simulink model "Satellite_formation_control_stable_consensus"  (R2022b)
settings: Solver=VariableStepAuto  StartTime=0.0  StopTime=500  RelTol=1e-3
values from neighbouring files (symbols this model uses):
  Am = kron(eye(N),A)    [Robust_consensus.m]    (also in Robust_consensus_S_procedure.m = blkdiag(A,(1+delta2)*A, (1+delta3)*A, (1+delta4)*A, (1+delta; Robust_consensus_against_model_uncertainty.m = blkdiag(A,A+Delta2, A+Delta3, A+Delta4, A+Delta5, A+Delta6); Stable_Consensus.m; alpha_stability.m = blkdiag(A,A+Delta2, A+Delta3, A+Delta4, A+Delta5, A+Delta6))
  Bm = kron(eye(N),B)    [Robust_consensus.m]    (also in Robust_consensus_S_procedure.m; Robust_consensus_against_model_uncertainty.m; Stable_Consensus.m; alpha_stability.m)
  Cm = kron(eye(N),C)    [output_feedback_formation_control.m]
  Km = kron(L,-c*B*K)    [Robust_consensus.m]    (also in Robust_consensus_S_procedure.m; Robust_consensus_against_model_uncertainty.m; Stable_Consensus.m; alpha_stability.m = kron(L,c*B*K))
  x0 = [x1_0 ... (first row only)    [Robust_consensus.m]    (also in Robust_consensus_S_procedure.m; Robust_consensus_against_model_uncertainty.m; Stable_Consensus.m; alpha_stability.m)
  x1_0 = [0 500 866*sqrt(3) 1.5 0 0].'    [Robust_consensus.m]    (also in Robust_consensus_S_procedure.m; Robust_consensus_against_model_uncertainty.m; Stable_Consensus.m; alpha_stability.m)
  xd = [x1d ... (first row only)    [Robust_consensus.m]    (also in Robust_consensus_S_procedure.m; Robust_consensus_against_model_uncertainty.m; Stable_Consensus.m; alpha_stability.m)
settings Model: Creator=yu zheng  LastModifiedBy=Abelb
settings SolverCC: AlgebraicLoopSolver=TrustRegion
settings DebuggingCC: UnconnectedInputMsg=warning  UnconnectedOutputMsg=warning  UnconnectedLineMsg=warning  SFMachineParentedDataDiag=warning
settings ModelReferenceCC: EnableRefExpFcnMdlSchedulingChecks=on
settings RTWCC: DLArmComputeVersion=19.05

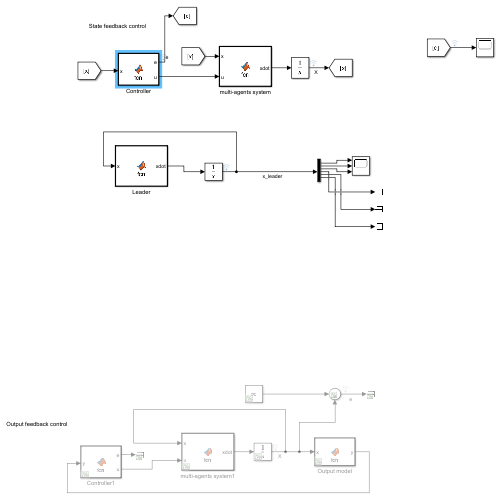
[thumbnail: Simulink's stored preview of the top-level diagram]
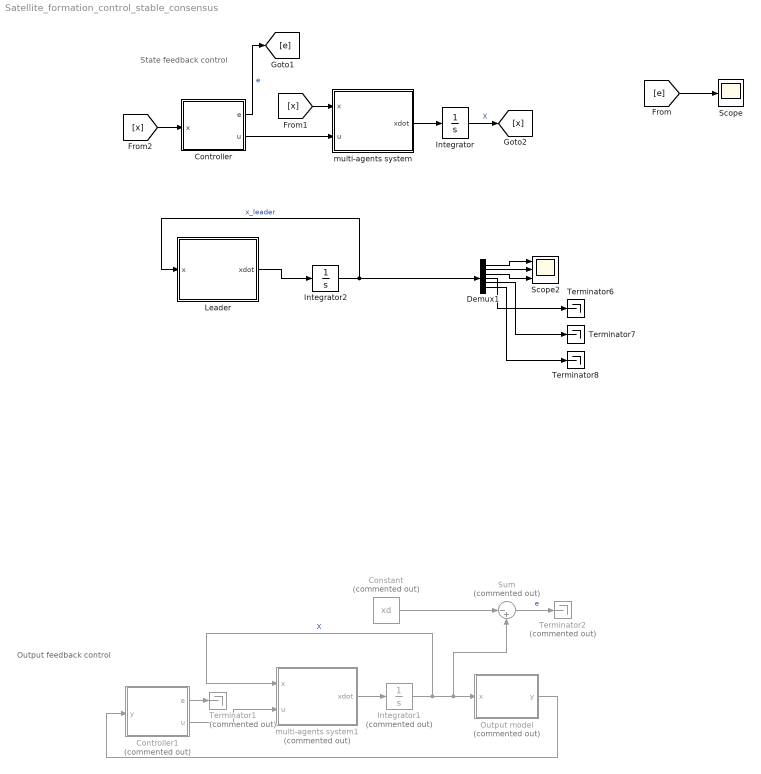
== system Satellite_formation_control_stable_consensus ==
  note: State feedback control
  note: Output feedback control
  Constant : Constant  Commented=on  Value=xd
  Controller : MATLAB Function  TreatAsAtomicUnit=on
  Controller1 : MATLAB Function  Commented=on  TreatAsAtomicUnit=on
  Demux1 : Demux  Outputs=6
  Integrator : Integrator  InitialCondition=x0
  Integrator1 : Integrator  Commented=on  InitialCondition=x0
  Integrator2 : Integrator  InitialCondition=x1_0
  Leader : MATLAB Function  TreatAsAtomicUnit=on
  Output model : MATLAB Function  Commented=on  TreatAsAtomicUnit=on
  Scope : Scope
  Scope2 : Scope  NumInputPorts=3
  Sum : Sum  Commented=on  Inputs=|-+
  Terminator1 : Terminator  Commented=on
  Terminator2 : Terminator  Commented=on
  Terminator6 : Terminator
  Terminator7 : Terminator
  Terminator8 : Terminator
  multi-agents system : MATLAB Function  TreatAsAtomicUnit=on
  multi-agents system1 : MATLAB Function  Commented=on  TreatAsAtomicUnit=on
  wires:
  multi-agents system/1(xdot) -> Integrator/1
  Integrator/1 -> [x]  "X"
  Controller/2(u) -> multi-agents system/2(u)
  Controller/1(e) -> [e]  "e"
  multi-agents system1/1(xdot) -> Integrator1/1
  Controller1/2(u) -> multi-agents system1/2(u)
  Integrator1/1 -> Sum/2, Output model/1(x), multi-agents system1/1(x)  "X"
  Controller1/1(e) -> Terminator1/1
  Output model/1(y) -> Controller1/1(y)
  Constant/1 -> Sum/1
  Sum/1 -> Terminator2/1  "e"
  Leader/1(xdot) -> Integrator2/1
  Demux1/4 -> Terminator6/1
  Demux1/1 -> Scope2/1
  Demux1/2 -> Scope2/2
  Integrator2/1 -> Leader/1(x), Demux1/1  "x_leader"
  Demux1/3 -> Scope2/3
  Demux1/6 -> Terminator8/1
  Demux1/5 -> Terminator7/1
  [x] -> multi-agents system/1(x)
  [x] -> Controller/1(x)
  [e] -> Scope/1

== matlab function Satellite_formation_control_stable_consensus/Controller ==
  data: e output; x input; u output; xd parameter; Km parameter
function [e,u] = fcn(x,xd,Km)

% x1 = x(1:n);
% x2 = x(n+1:2*n);
% x3 = x(2*n+1:3*n);
% x4 = x(3*n+1:4*n);
% x5 = x(4*n+1:5*n);
% x6 = x(5*n+1:6*n);

% e = Um*(x-xd);
e = x-xd;
u = Km*(x-xd);
u(1:6)=zeros(6,1);

== matlab function Satellite_formation_control_stable_consensus/multi-agents system ==
  data: x input; u input; xdot output; Am parameter
function xdot = fcn(x,u,Am)


xdot = Am*x +u ;

== matlab function Satellite_formation_control_stable_consensus/Controller1 ==
  data: e output; y input; u output; xd parameter; Km parameter; Am parameter; Cm parameter
function [e,u] = fcn(y,xd,Km,Am,Cm)

% x1 = x(1:n);
% x2 = x(n+1:2*n);
% x3 = x(2*n+1:3*n);
% x4 = x(3*n+1:4*n);
% x5 = x(4*n+1:5*n);
% x6 = x(5*n+1:6*n);

e = y-Cm*xd;
u = -Am*xd + Km*e;
u(1:6)=zeros(6,1);

== matlab function Satellite_formation_control_stable_consensus/multi-agents system1 ==
  data: x input; u input; xdot output; Am parameter; Bm parameter
function xdot = fcn(x,u,Am, Bm)

xdot = Am*x +u;

== matlab function Satellite_formation_control_stable_consensus/Output model ==
  data: x input; y output; Cm parameter
function y = fcn(x,Cm)

y = Cm*x;

== matlab function Satellite_formation_control_stable_consensus/Leader ==
  data: x input; xdot output; A parameter
function xdot = fcn(x, A)

n = size(A,1);
xdot = A*x ;
